simulink model "modele3"  (R2026a)
settings: Solver=VariableStepAuto
values from neighbouring files (symbols this model uses):
  params = [m, f, Yg, I, Lg, rho, S, Fx, Fy]    [init_params.m]
settings Model: Creator=floberg  LastModifiedBy=floberg

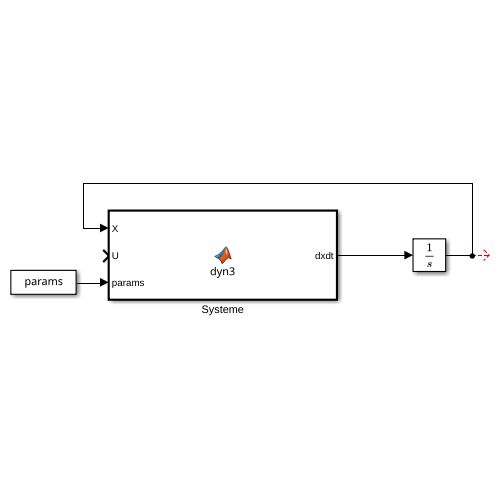
[thumbnail: Simulink's stored preview of the top-level diagram]
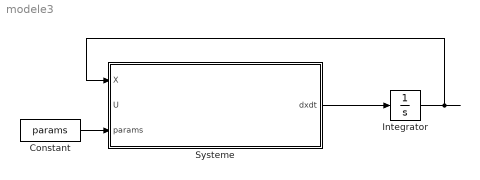
== system modele3 ==
  Constant : Constant  Value=params
  Integrator : Integrator
  Systeme : MATLAB Function  TreatAsAtomicUnit=on
  wires:
  Systeme/1(dxdt) -> Integrator/1
  Integrator/1 -> Systeme/1(X)
  Constant/1 -> Systeme/3(params)

== matlab function modele3/Systeme ==
  data: X input size=[6 1]; dxdt output size=[6 1]; U input size=[2 1]; params input size=[9 1]
function dxdt = dyn3(X, U, params)

phi = X(3);
u   = X(4);   % vitesse longitudinale dans Rb
v   = X(5);   % vitesse latérale dans Rb
r   = X(6);   % vitesse de lacet

T     = U(1);
theta = U(2);

m   = params(1);
Yg  = params(3);
I   = params(4);
Lg  = params(5);
rho = params(6);
S   = params(7);
Fx  = params(8);
Fy  = params(9);

% Angles
alpha = atan2(v, u);   % angle d'incidence sur le bateau
beta  = alpha - theta; % angle d'incidence sur la gouverne

cphi = cos(phi);
sphi = sin(phi);

% Matrice de rotation de Rb dans R0
R = [cphi -sphi; sphi cphi];

% Vitesses
V = R*[u; v]; % [vx; vy]
V_norm = sqrt(u^2 + v^2);

% Forces
Fg = rho*S*sin(2*beta)*V_norm^2; % Force de gouverne (Norme)
FT_vec = T*[1; 0];  % Force de gouverne dans Rb
Fg_vec = Fg*[sin(theta); -cos(theta)];
Ff_vec = [-Fx*u*abs(u); -Fy*v*abs(v)];

% Acceleration
a = (FT_vec + Fg_vec + Ff_vec)/m + [v*r; u*r];

% Equations d'etat
dx   = V(1);
dy   = V(2);
dphi = r;
du   = a(1);
dv   = a(2);
dr   = (Fg * Lg * cos(theta) - Yg * r) / I;

dxdt = [dx; dy; dphi; du; dv; dr];
end
